simulink model "diagrama_bloques"  (R2021a)
settings: Solver=VariableStepAuto  StartTime=0.0  StopTime=10.0  RelTol=1e-3
libraries: dspadpt3 x1
settings Model: Creator=Irek  LastModifiedBy=Irek

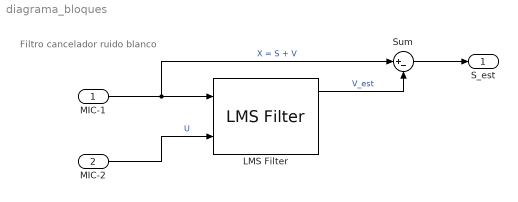
== system diagrama_bloques ==
  note: Filtro cancelador ruido blanco
  MIC-1 : Inport
  MIC-2 : Inport  Port=2
  LMS Filter : dspadpt3/LMS Filter  Algo=LMS  L=32  stepflag=Dialog  mu=0.1  leakage=1.0  ic=0  Adapt=off  resetflag=None  weights=on  addnparflag=off  roundingMode=Floor  overflowMode=off  secondCoeffMode=Binary point scaling  secondCoeffWordLength=2  secondCoeffFracLength=15  prodOutput2Mode=Binary point scaling  prodOutput2FracLength=20  prodOutput3Mode=Binary point scaling  prodOutput3FracLength=20  prodOutput4Mode=Binary point scaling  prodOutput4FracLength=20  quotientMode=Binary point scaling  quotientFracLength=20  accum2Mode=Binary point scaling  accum2FracLength=20
      settings: SourceProductBaseCode=DS
  Sum : Sum  Inputs=|+-
  S_est : Outport
  wires:
  MIC-1/1 -> Sum/1, LMS Filter/1  "X = S + V"
  MIC-2/1 -> LMS Filter/2  "U"
  LMS Filter/1 -> Sum/2  "V_est"
  Sum/1 -> S_est/1
